simulink model "Courant_2021A"  (R2021a)
settings: Solver=VariableStepAuto  StartTime=0.0  StopTime=0.2  FixedStep=0.001  RelTol=1e-3
values from neighbouring files (symbols this model uses):
  LL = .115    (= 0.115)    [Constante_NL.m]
  RR = 3.6    [Constante_NL.m]
settings Model: Creator=dupa1607  LastModifiedBy=alexi
settings SolverCC: AlgebraicLoopSolver=TrustRegion
settings DebuggingCC: SFMachineParentedDataDiag=warning

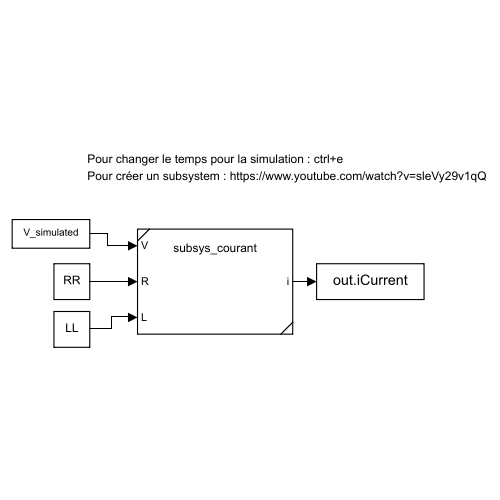
[thumbnail: Simulink's stored preview of the top-level diagram]
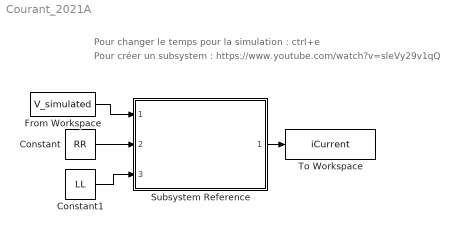
== system Courant_2021A ==
  note: Pour créer un subsystem : https://www.youtube.com/watch?v=sleVy29v1qQ
  note: Pour changer le temps pour la simulation : ctrl+e
  Constant : Constant  Value=RR
  Constant1 : Constant  Value=LL
  From Workspace : FromWorkspace  VariableName=V_simulated
  Subsystem Reference : Subsystem  ReferencedSubsystem=subsys_courant
  To Workspace : ToWorkspace  VariableName=iCurrent  SaveFormat=Timeseries  SampleTime=-1
  wires:
  Subsystem Reference/1 -> To Workspace/1
  From Workspace/1 -> Subsystem Reference/1
  Constant/1 -> Subsystem Reference/2
  Constant1/1 -> Subsystem Reference/3
